simulink model "jieyue"  (R2012b)
settings: Solver=ode45  StartTime=0.0  StopTime=10  MaxStep=0.01  RelTol=1e-3
settings Model: Creator=Administrator  LastModifiedBy=Administrator

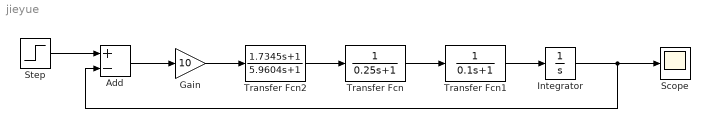
== system jieyue ==
  Add : Sum  Inputs=+-
  Gain : Gain  Gain=10
  Integrator : Integrator
  Scope : Scope
  Step : Step  SampleTime=0
  Transfer Fcn : TransferFcn  Denominator=[0.25 1]
  Transfer Fcn1 : TransferFcn  Denominator=[0.1 1]
  Transfer Fcn2 : TransferFcn  Numerator=[1.7345 1]  Denominator=[5.9604 1]
  wires:
  Gain/1 -> Transfer Fcn2/1
  Transfer Fcn/1 -> Transfer Fcn1/1
  Step/1 -> Add/1
  Add/1 -> Gain/1
  Integrator/1 -> Add/2, Scope/1
  Transfer Fcn1/1 -> Integrator/1
  Transfer Fcn2/1 -> Transfer Fcn/1
